simulink model "case_1_leadcar_stationary_egocar_move25a"  (R2025a)
settings: Solver=VariableStepAuto  StartTime=0.0  StopTime=10.0  RelTol=1e-3
settings Model: Creator=jdcjd  LastModifiedBy=sanborkl

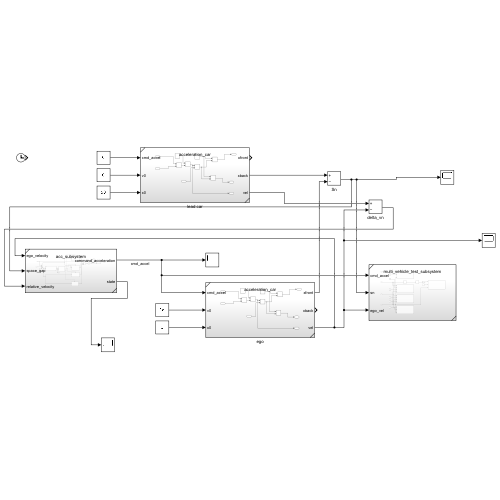
[thumbnail: Simulink's stored preview of the top-level diagram]
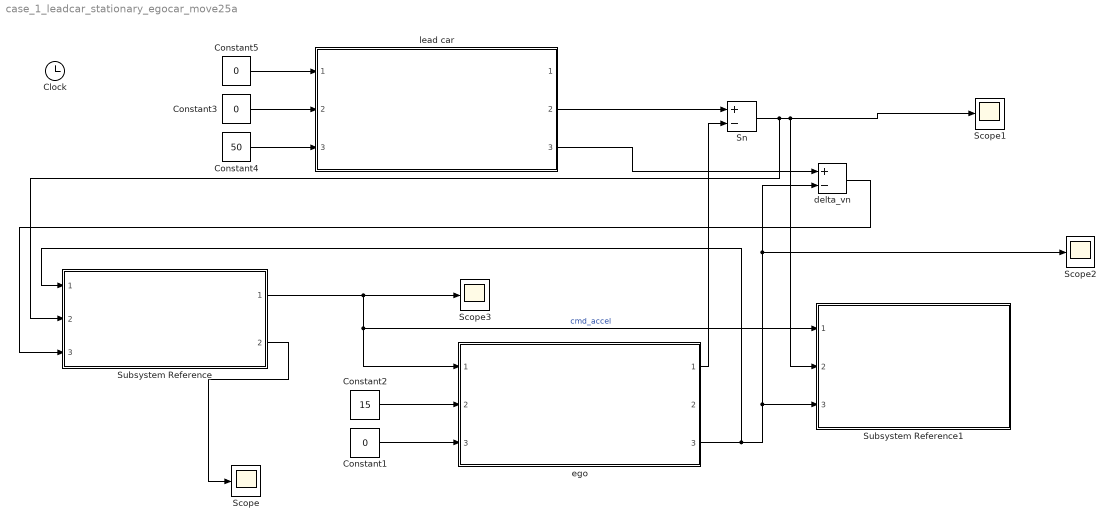
== system case_1_leadcar_stationary_egocar_move25a ==
  Clock : Clock
  Constant1 : Constant  Value=0
  Constant2 : Constant  Value=15
  Constant3 : Constant  Value=0
  Constant4 : Constant  Value=50
  Constant5 : Constant  Value=0
  Scope{,1..3} (4 alike) : Scope
      Scope1 settings: ActiveDisplayYMinimum=-20.738899101530652  ActiveDisplayYMaximum=47.901076576046918
      Scope2 settings: ActiveDisplayYMinimum=-2.0348114284014764  ActiveDisplayYMaximum=18.313302855613291  DataLoggingVariableName=ScopeData2
      Scope3 settings: ActiveDisplayYMinimum=-6.885608060883305  ActiveDisplayYMaximum=2.2766223789446967  DataLoggingVariableName=ScopeData3
  Sn : Sum  Inputs=+-
  Subsystem Reference : Subsystem  ReferencedSubsystem=acc_subsystem
  Subsystem Reference1 : Subsystem  ReferencedSubsystem=multi_vehicle_test_subsystem
  delta_vn : Sum  Inputs=+-
  ego : Subsystem  ReferencedSubsystem=acceleration_car
  lead car : Subsystem  ReferencedSubsystem=acceleration_car
  wires:
  Constant5/1 -> lead car/1
  Constant3/1 -> lead car/2
  Constant4/1 -> lead car/3
  Constant2/1 -> ego/2
  Constant1/1 -> ego/3
  Subsystem Reference/1 -> Scope3/1, ego/1, Subsystem Reference1/1  "cmd_accel"
  ego/1 -> Sn/2
  lead car/2 -> Sn/1
  lead car/3 -> delta_vn/1
  delta_vn/1 -> Subsystem Reference/3
  Sn/1 -> Subsystem Reference1/2, Scope1/1, Subsystem Reference/2
  Subsystem Reference/2 -> Scope/1
  ego/3 -> Subsystem Reference/1, Scope2/1, delta_vn/2, Subsystem Reference1/3
